simulink model "Dynamic_Compensator"  (R2025b)
settings: Solver=VariableStepAuto  StartTime=0.0  StopTime=500  RelTol=1e-3
values from neighbouring files (symbols this model uses):
  AL = A-L*C    [fase1.m]
  BL = [Bu L]    [fase1.m]
  C = [1, 0, 0]    [fase1.m]
  CL = eye(size(A))    [fase1.m]
  DL = zeros(size(A,1),2)    [fase1.m]
  K = place(A, Bu, poles_SSF)    [fase1.m]
  yeq = xeq(1,:)    [fase1.m]
undefined symbols (not defined in the file or in its folder): ueq
settings Model: Creator=Rika  LastModifiedBy=Rika

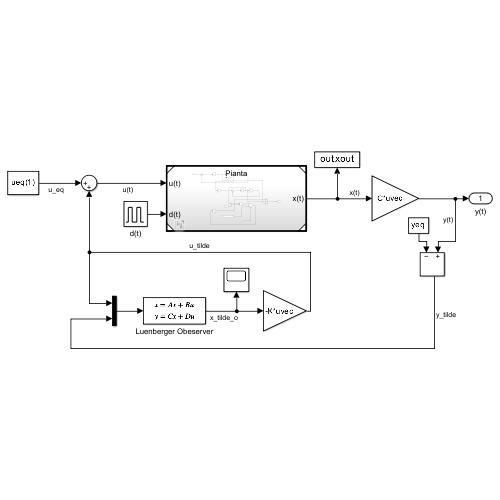
[thumbnail: Simulink's stored preview of the top-level diagram]
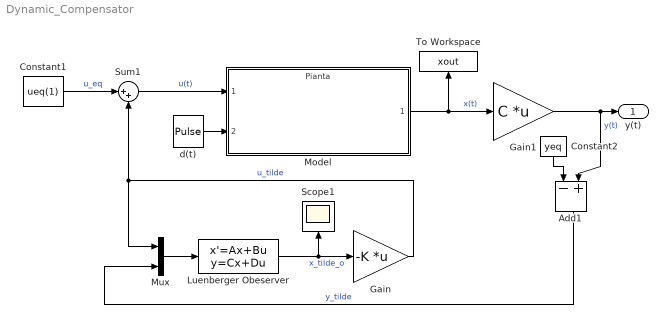
== system Dynamic_Compensator ==
  Add1 : Sum  Inputs=-+
  Constant1 : Constant  Value=ueq(1)
  Constant2 : Constant  Value=yeq
  Gain : Gain  Gain=-K  Multiplication=Matrix(K*u) (u vector)
  Gain1 : Gain  Gain=C  Multiplication=Matrix(K*u) (u vector)
  Luenberger Obeserver : StateSpace  A=AL  B=BL  C=CL  D=DL  InitialCondition=0
  Model : ModelReference  ModelNameDialog=Pianta.slx  SimulationMode=Normal  ModelReferenceVersion=1.16
  Mux : Mux  Inputs=2
  Scope1 : Scope
      settings: ActiveDisplayYMinimum=-1  ActiveDisplayYMaximum=1
  Sum1 : Sum  Inputs=|++
  To Workspace : ToWorkspace  VariableName=xout  SaveFormat=Timeseries  SampleTime=-1
  d(t) : DiscretePulseGenerator  PulseType=Time based  Amplitude=10  Period=1000  PulseWidth=3  PhaseDelay=10
  y(t) : Outport
  wires:
  Model/1 -> Gain1/1, To Workspace/1  "x(t)"
  Constant1/1 -> Sum1/1  "u_eq"
  Gain1/1 -> Add1/2, y(t)/1  "y(t)"
  Gain/1 -> Mux/1, Sum1/2  "u_tilde"
  d(t)/1 -> Model/2
  Sum1/1 -> Model/1  "u(t)"
  Luenberger Obeserver/1 -> Scope1/1, Gain/1  "x_tilde_o"
  Mux/1 -> Luenberger Obeserver/1
  Constant2/1 -> Add1/1
  Add1/1 -> Mux/2  "y_tilde"
